simulink library "Driveshaft_Assembly_None"  (R2022a)
settings: Solver=VariableStepAuto  StartTime=0.0  StopTime=10.0  RelTol=1e-3
libraries: Driveshaft_Utilities x1, sm_lib x1
Description:
  | Component of Simscape Vehicle Templates Library
  | 
  | Copyright 2018-2024 The MathWorks, Inc.
settings Model: Creator=smiller  LastModifiedBy=smiller
settings SolverCC: AlgebraicLoopSolver=TrustRegion
settings DataIOCC: ReturnWorkspaceOutputs=off
settings DebuggingCC: UnconnectedInputMsg=warning  UnconnectedOutputMsg=warning  UnconnectedLineMsg=warning  SFMachineParentedDataDiag=warning  ArithmeticOperatorsInVariantConditions=warning
settings SFSimCC: CustomCodeUndefinedFunction=UseInterfaceOnly
settings RTWCC: DLArmComputeVersion=19.05

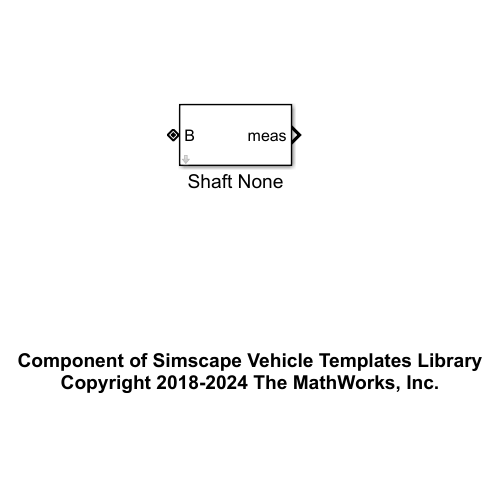
[thumbnail: Simulink's stored preview of the top-level diagram]
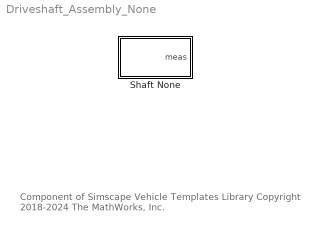
== system Driveshaft_Assembly_None ==
  note: Component of Simscape Vehicle Templates Library
      | Copyright 2018-2024 The MathWorks, Inc.
  Shaft None : Subsystem  VariantControl=Shaft1D  mask(Driveshaft Assembly (1D)){}
      mask help: Models a shaft as a 1D mechanical connection.

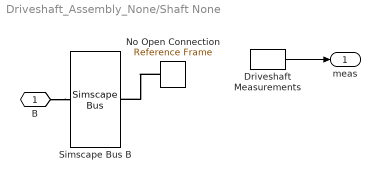
== system Driveshaft_Assembly_None/Shaft None ==
  Driveshaft Measurements : Driveshaft_Utilities/Driveshaft Measurements  SystemSampleTime=-1  VariantActivationTime=update diagram  Latency=0  AutoFrameSizeCalculation=off
  No Open Connection : sm_lib/Frames and Transforms/Reference Frame
  Simscape Bus B : SimscapeBus  HierarchyStrings=AxleIn
  B : PMIOPort  Side=Left
  meas : Outport  VectorParamsAs1DForOutWhenUnconnected=off
  wires:
  Driveshaft Measurements/1 -> meas/1
  connections:
  No Open Connection/RConn1 -- Simscape Bus B/LConn1
  B/RConn1 -- Simscape Bus B/RConn1
